simulink model "sim_PD"  (R2023a)
settings: Solver=VariableStepAuto  StartTime=0.0  StopTime=20  RelTol=1e-3
undefined symbols (not defined in the file): Beff, Jeff, Kd, Km_R, Kp, m, r
libraries: lib_robotRP_new x5
settings Model: Creator=gbl3344a  LastModifiedBy=gbl3344a

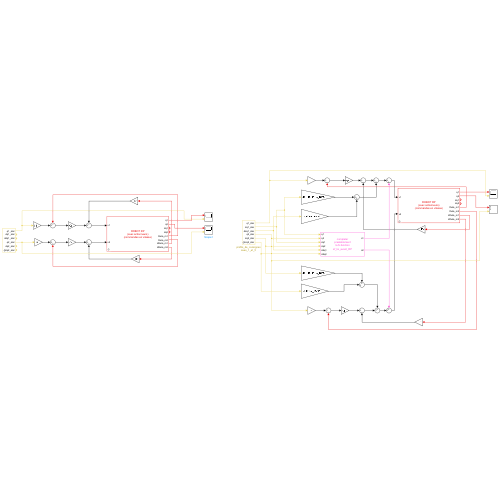
[thumbnail: Simulink's stored preview of the top-level diagram]
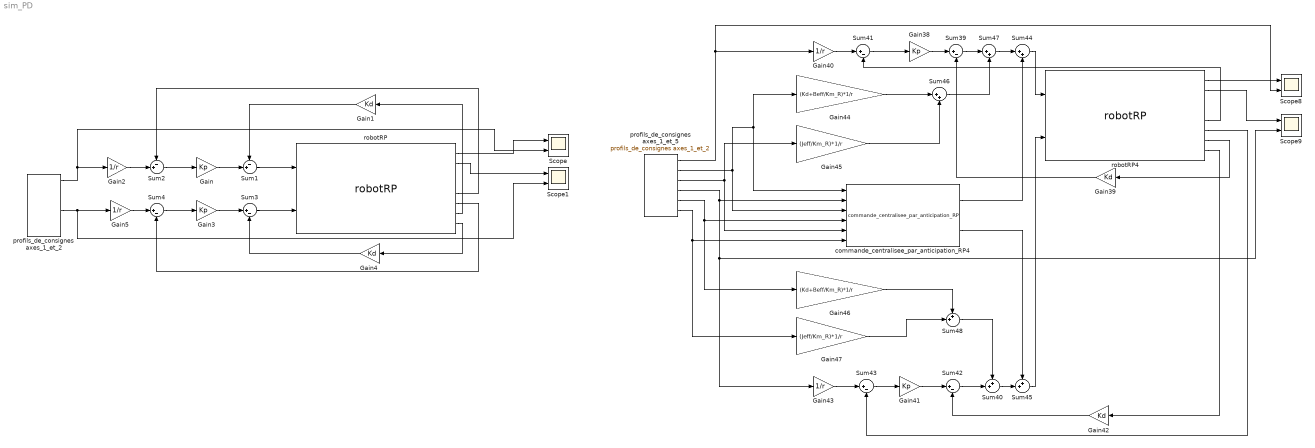
== system sim_PD ==
  Gain{,3,38,41} (4 alike) : Gain  Gain=Kp
  Gain{1,4,39,42} (4 alike) : Gain  Gain=Kd
  Gain{2,5,40,43} (4 alike) : Gain  Gain=1/r
  Gain44 : Gain  Gain=(Kd+Beff/Km_R)*1/r
  Gain45 : Gain  Gain=(Jeff/Km_R)*1/r
  Gain46 : Gain  Gain=(Kd+Beff/Km_R)*1/r
  Gain47 : Gain  Gain=(Jeff/Km_R)*1/r
  Scope{,1,8..9} (4 alike) : Scope  NumInputPorts=2
  Sum1 : Sum  Inputs=-+|
  Sum2 : Sum  Inputs=-+|
  Sum{3..4,39,41..43} (6 alike) : Sum  Inputs=|+-
  Sum40 : Sum  Inputs=++|
  Sum44 : Sum  Inputs=|++
  Sum45 : Sum  Inputs=++|
  Sum46 : Sum  Inputs=|++
  Sum47 : Sum  Inputs=|++
  Sum48 : Sum  Inputs=++|
  commande_centralisee_par_anticipation_RP4 : lib_robotRP_new/commande_centralisee_par_anticipation_RP  SystemSampleTime=-1  VariantActivationTime=update diagram  Latency=0  AutoFrameSizeCalculation=off
  profils_de_consignes axes_1_et_2 : lib_robotRP_new/profils_de_consignes axes_1_et_2
  profils_de_consignes axes_1_et_5 : lib_robotRP_new/profils_de_consignes axes_1_et_2
  robotRP : lib_robotRP_new/robotRP  vecteur_theta_dtheta_initial=[0 ; 0.5/r ; 0 ; 0]  m=m  gX=0  gY=0  F1=0  F2=0  H1=0  H2=0  Km_sur_R=Km_R  Jm=Jm  Beff=Beff  r=r
  robotRP4 : lib_robotRP_new/robotRP  vecteur_theta_dtheta_initial=[0 ; 0.5/r ; 0 ; 0]  m=m  gX=0  gY=0  F1=0  F2=0  H1=0  H2=0  Km_sur_R=Km_R  Jm=Jm  Beff=Beff  r=r
  wires:
  Sum2/1 -> Gain/1
  profils_de_consignes axes_1_et_2/1 -> Scope/2, Gain2/1
  Gain3/1 -> Sum3/1
  Gain4/1 -> Sum3/2
  Gain5/1 -> Sum4/1
  Sum4/1 -> Gain3/1
  profils_de_consignes axes_1_et_2/4 -> Scope1/2, Gain5/1
  robotRP/6 -> Sum4/2
  robotRP/8 -> Gain4/1
  robotRP/7 -> Gain1/1
  robotRP/2 -> Scope1/1
  robotRP/1 -> Scope/1
  Sum1/1 -> robotRP/1
  Sum46/1 -> Sum47/2
  Sum39/1 -> Sum47/1
  Gain46/1 -> Sum48/1
  Gain47/1 -> Sum48/2
  Gain45/1 -> Sum46/2
  profils_de_consignes axes_1_et_5/6 -> commande_centralisee_par_anticipation_RP4/6, Gain47/1
  Sum47/1 -> Sum44/1
  profils_de_consignes axes_1_et_5/3 -> Gain45/1, commande_centralisee_par_anticipation_RP4/5
  Sum45/1 -> robotRP4/2
  robotRP4/2 -> Scope9/1
  robotRP4/5 -> Sum41/2
  robotRP4/6 -> Sum43/2
  Gain44/1 -> Sum46/1
  Sum43/1 -> Gain41/1
  profils_de_consignes axes_1_et_5/5 -> commande_centralisee_par_anticipation_RP4/4, Gain46/1
  profils_de_consignes axes_1_et_5/4 -> commande_centralisee_par_anticipation_RP4/2, Gain43/1, Scope9/2
  robotRP4/1 -> Scope8/1
  robotRP4/8 -> Gain42/1
  robotRP4/7 -> Gain39/1
  profils_de_consignes axes_1_et_5/1 -> Gain40/1, Scope8/2
  Gain41/1 -> Sum42/1
  Gain38/1 -> Sum39/1
  profils_de_consignes axes_1_et_5/2 -> commande_centralisee_par_anticipation_RP4/1, Gain44/1, commande_centralisee_par_anticipation_RP4/3
  Gain43/1 -> Sum43/1
  Gain39/1 -> Sum39/2
  Sum41/1 -> Gain38/1
  Gain40/1 -> Sum41/1
  Sum44/1 -> robotRP4/1
  commande_centralisee_par_anticipation_RP4/1 -> Sum44/2
  Gain42/1 -> Sum42/2
  Sum3/1 -> robotRP/2
  Gain/1 -> Sum1/2
  Gain1/1 -> Sum1/1
  robotRP/5 -> Sum2/1
  Gain2/1 -> Sum2/2
  Sum48/1 -> Sum40/1
  Sum42/1 -> Sum40/2
  commande_centralisee_par_anticipation_RP4/2 -> Sum45/1
  Sum40/1 -> Sum45/2
